simulink subsystem "controller_BA"  (R2023b)
settings: Solver=VariableStepAuto  StartTime=0.0  StopTime=10.0  RelTol=1e-3
settings Model: Creator=ricfe  LastModifiedBy=ricfe

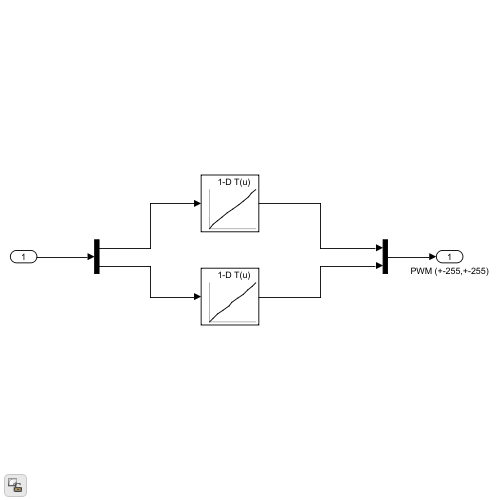
[thumbnail: Simulink's stored preview of the top-level diagram]
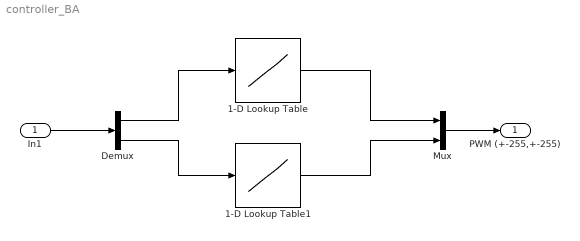
== system controller_BA ==
  In1 : Inport
  1-D Lookup Table : Lookup_n-D  NumberOfTableDimensions=1  BreakpointsForDimension1=[-0.511085510253906 -0.438068389892578 -0.335855484008789 -0.233636856079102 -0.116818785667419 0 0.131416320800781 0.233634948730469 0.350456237792969 0.423469543457031 0.511077880859375]  Table=[-254 -200.660049438477 -151.130004882813 -100.32999420166 -49.5300445556641 0 51 99.4500274658203 150.450012207031 200.175018310547 249.900009155273]  InternalRulePriority=Speed  RndMeth=Simplest
  1-D Lookup Table1 : Lookup_n-D  NumberOfTableDimensions=1  BreakpointsForDimension1=[-0.481880187988281 -0.40887451171875 -0.306648254394531 -0.204429626464844 -0.0730133056640625 0 0.131416320800781 0.233642578125 0.335861206054688 0.4234619140625 0.496482849121094]  Table=[-250.189971923828 -200.65998840332 -149.859985351563 -100.32999420166 -49.5299835205078 0 49.724983215332 99.4500274658203 150.450012207031 200.175018310547 249.900009155273]  InternalRulePriority=Speed  RndMeth=Simplest
  Demux : Demux  Outputs=2
  Mux : Mux  Inputs=2
  PWM (+-255,+-255) : Outport
  wires:
  Demux/1 -> 1-D Lookup Table/1
  Demux/2 -> 1-D Lookup Table1/1
  1-D Lookup Table1/1 -> Mux/2
  1-D Lookup Table/1 -> Mux/1
  Mux/1 -> PWM (+-255,+-255)/1
  In1/1 -> Demux/1
